simulink model "tensegrity_Val_like_sim"  (R2022b)
settings: Solver=ode15s  StartTime=0.0  StopTime=10  MaxStep=0.001  RelTol=1e-3
InitFcn:
  | tensegrity_Val_like;
values from neighbouring files (symbols this model uses):
  a = 0.015    [parameters.m]
  bar_or_cable = 1    [parameters.m]
  bb = 100    [parameters.m]
  F1 = [pos1(1), pos1(2), pos1(3)]    [parameters.m]
  F2 = [pos1(1)+dist, pos1(2), pos1(3)]    [parameters.m]
  F3 = [pos1(1)+dist/2, pos1(2)+dist, pos1(3)]    [parameters.m]
  F4 = [pos2(1), pos2(2), pos2(3)]    [parameters.m]
  F5 = [pos2(1)+dist, pos2(2), pos2(3)]    [parameters.m]
  F6 = [pos2(1)+dist/2, pos2(2)+dist, pos2(3)]    [parameters.m]
  F7 = [pos3(1), pos3(2), pos3(3)]    [parameters.m]
  F8 = [pos3(1)+dist, pos3(2), pos3(3)]    [parameters.m]
  F9 = [pos3(1)+dist/2, pos3(2)+dist, pos3(3)]    [parameters.m]
  kk = 5e4    (= 50000)    [parameters.m]
  l = [0.08 0.08 0.08 0.15]'    [parameters.m]
  lf = 0.05*ones(9, 1)    [parameters.m]
undefined symbols (not defined in the file or in its folder): A1, lengths_0, X, Y, Z
libraries: sm_lib x34, nesl_utility x31
(part 2 of 2)

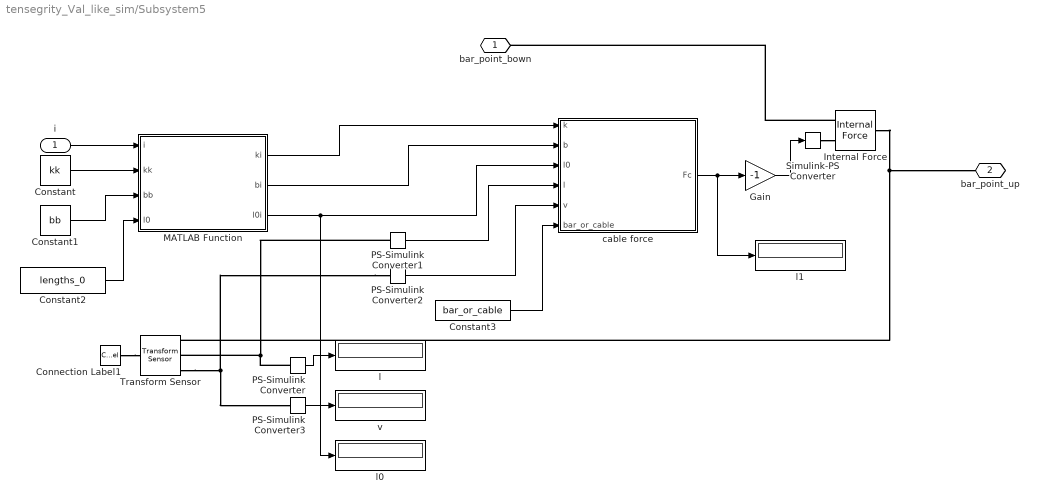
== system tensegrity_Val_like_sim/Subsystem5 ==
  i : Inport
  Connection Label1 : ConnectionLabel  Label=base_frame
  Constant : Constant  Value=kk
  Constant1 : Constant  Value=bb
  Constant2 : Constant  Value=lengths_0
  Constant3 : Constant  Value=bar_or_cable
  Gain : Gain  Gain=-1
  Internal Force : sm_lib/Forces and Torques/Internal Force
  MATLAB Function : MATLAB Function  TreatAsAtomicUnit=on
  PS-Simulink Converter{,1..3} (4 alike) : nesl_utility/PS-Simulink Converter  PhysicalDomain=network_engine_domain  SubClassName=ps_output  LeftPortType=input  RightPortType=output  PseudoPeriodic=off  Frequencies=[]  VectorFormat=inherit  Unit=inherit  AffineConversion=off
  Simulink-PS Converter : nesl_utility/Simulink-PS Converter  PhysicalDomain=network_engine_domain  SubClassName=ps_input  LeftPortType=input  RightPortType=output  PseudoPeriodic=off  Frequencies=[]  NoiseDistribution=none  NoiseParameters=[]  Unit=1  AffineConversion=off  FilteringAndDerivatives=provide  SimscapeFilterOrder=1  InputFilterTimeConstant=0.001  UdotUserProvided=0
  Transform Sensor : sm_lib/Frames and Transforms/Transform Sensor  MeasurementFrame=World  SenseAngle=off  SenseAxis=off  SenseQ=off  SenseR=off  SenseRotationSequence=off  RotationSequence=XYX  SenseOmegaX=off  SenseOmegaY=off  SenseOmegaZ=off  SenseQDot=off  SenseRDot=off  SenseAlphaX=off  SenseAlphaY=off  SenseAlphaZ=off  SenseQDDot=off  SenseRDDot=off  SenseX=off  SenseY=off  SenseZ=off  SenseRad=off  SenseAzim=off  SenseDist=on  SenseInc=off  SenseXDot=off  SenseYDot=off  SenseZDot=off  SenseRadDot=off  SenseAzimDot=off  SenseDistDot=on  SenseIncDot=off  SenseXDDot=off  SenseYDDot=off  SenseZDDot=off  SenseRadDDot=off  SenseAzimDDot=off  SenseDistDDot=off  SenseIncDDot=off
  cable force : MATLAB Function  TreatAsAtomicUnit=on
  l : Display
  l0 : Display
  l1 : Display
  v : Display
  bar_point_bown : PMIOPort  Side=Left
  bar_point_up : PMIOPort  Port=2  Side=Right
  wires:
  PS-Simulink Converter3/1 -> v/1
  PS-Simulink Converter2/1 -> cable force/5(v)
  Gain/1 -> Simulink-PS Converter/1
  Constant3/1 -> cable force/6(bar_or_cable)
  i/1 -> MATLAB Function/1(i)
  MATLAB Function/3(l0i) -> cable force/3(l0), l0/1
  PS-Simulink Converter1/1 -> cable force/4(l)
  MATLAB Function/1(ki) -> cable force/1(k)
  Constant/1 -> MATLAB Function/2(kk)
  Constant1/1 -> MATLAB Function/3(bb)
  MATLAB Function/2(bi) -> cable force/2(b)
  Constant2/1 -> MATLAB Function/4(l0)
  PS-Simulink Converter/1 -> l/1
  cable force/1(Fc) -> Gain/1, l1/1
  connections:
  PS-Simulink Converter2/LConn1 -- PS-Simulink Converter3/LConn1 -- Transform Sensor/RConn3
  Connection Label1/LConn1 -- Transform Sensor/LConn1
  Transform Sensor/RConn1 -- bar_point_up/RConn1 -- Internal Force/RConn1
  Simulink-PS Converter/RConn1 -- Internal Force/LConn2
  Transform Sensor/RConn2 -- PS-Simulink Converter1/LConn1 -- PS-Simulink Converter/LConn1
  Internal Force/LConn1 -- bar_point_bown/RConn1

== matlab function tensegrity_Val_like_sim/Subsystem4/MATLAB Function ==
  data: i input; ki output; kk input; bb input; l0 input; bi output; l0i output
function [ki, bi, l0i] = parameter_selection(i, kk, bb, l0)

l0i=l0(i);
ki=kk;
bi=bb;

== matlab function tensegrity_Val_like_sim/Subsystem/MATLAB Function ==
  data: i input; ki output; kk input; bb input; l0 input; bi output; l0i output
function [ki, bi, l0i] = parameter_selection(i, kk, bb, l0)

l0i=l0(i);
ki=kk;
bi=bb;

== matlab function tensegrity_Val_like_sim/Subsystem4/cable force ==
  data: k input; Fc output; b input; l0 input; l input; v input; bar_or_cable input
function Fc = fcn(k, b, l0, l, v, bar_or_cable)

Fc=0; %if not bar, but cable only

if(l>l0)
  Fc=k*(l-l0) + v*b;
end;

if(bar_or_cable==1) % if bar==1, the force can act in both directions
  Fc=k*(l-l0) + v*b;
end;

== matlab function tensegrity_Val_like_sim/Subsystem5/MATLAB Function ==
  data: i input; ki output; kk input; bb input; l0 input; bi output; l0i output
function [ki, bi, l0i] = parameter_selection(i, kk, bb, l0)

l0i=l0(i);
ki=kk;
bi=bb;

== matlab function tensegrity_Val_like_sim/Subsystem5/cable force ==
  data: k input; Fc output; b input; l0 input; l input; v input; bar_or_cable input
function Fc = fcn(k, b, l0, l, v, bar_or_cable)

Fc=0; %if not bar, but cable only

if(l>l0)
  Fc=k*(l-l0) + v*b;
end;

if(bar_or_cable==1) % if bar==1, the force can act in both directions
  Fc=k*(l-l0) + v*b;
end;

== matlab function tensegrity_Val_like_sim/Subsystem/cable force ==
  data: k input; Fc output; b input; l0 input; l input; v input; bar_or_cable input
function Fc = fcn(k, b, l0, l, v, bar_or_cable)

Fc=0; %if not bar, but cable only

if(l>l0)
  Fc=k*(l-l0) + b*v;
end;

if(bar_or_cable==1) % if bar==1, the force can act in both directions
  Fc=k*(l-l0) + v*b;
end;

== matlab function tensegrity_Val_like_sim/Subsystem1/MATLAB Function ==
  data: i input; ki output; kk input; bb input; l0 input; bi output; l0i output
function [ki, bi, l0i] = parameter_selection(i, kk, bb, l0)

l0i=l0(i);
ki=kk;
bi=bb;

== matlab function tensegrity_Val_like_sim/Subsystem1/cable force ==
  data: k input; Fc output; b input; l0 input; l input; v input; bar_or_cable input
function Fc = fcn(k, b, l0, l, v, bar_or_cable)

Fc=0; %if not bar, but cable only

if(l>l0)
  Fc=k*(l-l0) + v*b;
end;

if(bar_or_cable==1) % if bar==1, the force can act in both directions
  Fc=k*(l-l0) + v*b;
end;

== matlab function tensegrity_Val_like_sim/Subsystem2/MATLAB Function ==
  data: i input; ki output; kk input; bb input; l0 input; bi output; l0i output
function [ki, bi, l0i] = parameter_selection(i, kk, bb, l0)

l0i=l0(i);
ki=kk;
bi=bb;

== matlab function tensegrity_Val_like_sim/Subsystem2/cable force ==
  data: k input; Fc output; b input; l0 input; l input; v input; bar_or_cable input
function Fc = fcn(k, b, l0, l, v, bar_or_cable)

Fc=0; %if not bar, but cable only

if(l>l0)
  Fc=k*(l-l0) + v*b;
end;

if(bar_or_cable==1) % if bar==1, the force can act in both directions
  Fc=k*(l-l0) + v*b;
end;

== matlab function tensegrity_Val_like_sim/Subsystem3/MATLAB Function ==
  data: i input; ki output; kk input; bb input; l0 input; bi output; l0i output
function [ki, bi, l0i] = parameter_selection(i, kk, bb, l0)

l0i=l0(i);
ki=kk;
bi=bb;

== matlab function tensegrity_Val_like_sim/Subsystem3/cable force ==
  data: k input; Fc output; b input; l0 input; l input; v input; bar_or_cable input
function Fc = fcn(k, b, l0, l, v, bar_or_cable)

Fc=0; %if not bar, but cable only

if(l>l0)
  Fc=k*(l-l0) + v*b;
end;

if(bar_or_cable==1) % if bar==1, the force can act in both directions
  Fc=k*(l-l0) + v*b;
end;
